simulink model "LTI_equivalente"  (R2023a)
settings: Solver=VariableStepAuto  StartTime=0.0  StopTime=1  RelTol=1e-3
undefined symbols (not defined in the file or in its folder): b_eq, Cts, J_eq, k_l, lambda, Lq, Pp, r, Rs_ref, Rts
libraries: SignalEditorBlockLib x3
settings Model: Creator=tobip  LastModifiedBy=tobip

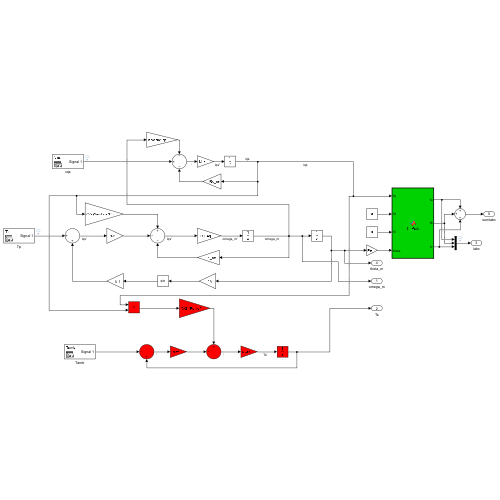
[thumbnail: Simulink's stored preview of the top-level diagram]
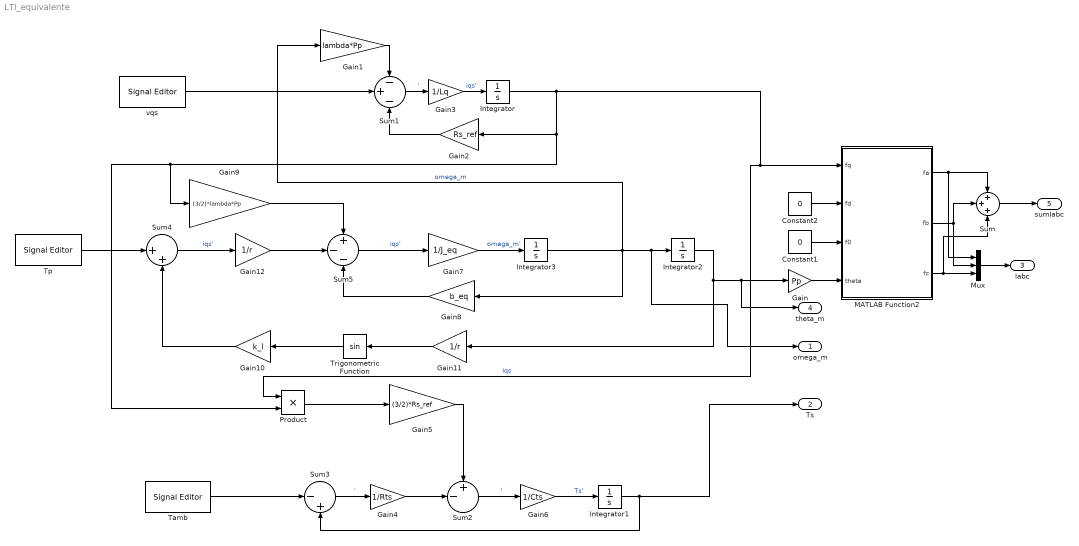
== system LTI_equivalente ==
  Constant1 : Constant  Value=0
  Constant2 : Constant  Value=0
  Gain : Gain  Gain=Pp
  Gain1 : Gain  Gain=lambda*Pp
  Gain10 : Gain  Gain=k_l
  Gain11 : Gain  Gain=1/r
  Gain12 : Gain  Gain=1/r
  Gain2 : Gain  Gain=Rs_ref
  Gain3 : Gain  Gain=1/Lq
  Gain4 : Gain  Gain=1/Rts
  Gain5 : Gain  Gain=(3/2)*Rs_ref
  Gain6 : Gain  Gain=1/Cts
  Gain7 : Gain  Gain=1/J_eq
  Gain8 : Gain  Gain=b_eq
  Gain9 : Gain  Gain=(3/2)*lambda*Pp
  Integrator{,1..3} (4 alike) : Integrator
  MATLAB Function2 : MATLAB Function  TreatAsAtomicUnit=on
  Mux : Mux  Inputs=3
  Product : Product
  Sum : Sum  Inputs=+++
  Sum1 : Sum  Inputs=-+-
  Sum2 : Sum  Inputs=+-|
  Sum3 : Sum  Inputs=|-+
  Sum4 : Sum  Inputs=|++
  Sum5 : Sum  Inputs=+--
  Tamb : SignalEditorBlockLib/Signal Editor  FileName=senal_Tamb.mat  ActiveScenario=Tamb  ActiveSignal=Constant  IsBus=off  OutputBusObjectStr=Bus: BusObject  SampleTime=0  Interpolate=off  ZeroCross=off  OutputAfterFinalValue=Setting to zero  Unit=inherit  PreserveSignalName=on  ApplySigPropsToAllScenarios=on
  Tp : SignalEditorBlockLib/Signal Editor  FileName=senal_Tp.mat  ActiveScenario=Tp  ActiveSignal=Pulse  IsBus=off  OutputBusObjectStr=Bus: BusObject  SampleTime=0  Interpolate=off  ZeroCross=off  OutputAfterFinalValue=Setting to zero  Unit=inherit  PreserveSignalName=on  ApplySigPropsToAllScenarios=on
  Trigonometric Function : Trigonometry
  vqs : SignalEditorBlockLib/Signal Editor  FileName=senal_vqs.mat  ActiveScenario=Vqs  ActiveSignal=Pulse  IsBus=off  OutputBusObjectStr=Bus: BusObject  SampleTime=0  Interpolate=off  ZeroCross=off  OutputAfterFinalValue=Setting to zero  Unit=inherit  PreserveSignalName=on  ApplySigPropsToAllScenarios=on
  omega_m : Outport
  Ts : Outport  Port=2
  Iabc : Outport  Port=3
  theta_m : Outport  Port=4
  sumIabc : Outport  Port=5
  wires:
  Integrator1/1 -> Ts/1, Sum3/2
  Integrator2/1 -> Gain/1, theta_m/1, Gain11/1
  Constant1/1 -> MATLAB Function2/3(f0)
  Gain/1 -> MATLAB Function2/4(theta)
  MATLAB Function2/1(fa) -> Sum/1, Mux/1
  MATLAB Function2/2(fb) -> Sum/2, Mux/2
  MATLAB Function2/3(fc) -> Mux/3, Sum/3
  Mux/1 -> Iabc/1
  Sum/1 -> sumIabc/1
  Constant2/1 -> MATLAB Function2/2(fd)
  Integrator/1 -> Gain2/1, Product/2, Gain9/1, Product/1, MATLAB Function2/1(fq)  "iqs"
  Gain1/1 -> Sum1/1
  vqs/1 -> Sum1/2
  Gain2/1 -> Sum1/3
  Sum1/1 -> Gain3/1  "'"
  Gain3/1 -> Integrator/1  "iqs'"
  Product/1 -> Gain5/1
  Tamb/1 -> Sum3/1
  Sum3/1 -> Gain4/1  "'"
  Sum2/1 -> Gain6/1  "'"
  Gain6/1 -> Integrator1/1  "Ts'"
  Gain4/1 -> Sum2/2
  Gain5/1 -> Sum2/1
  Gain11/1 -> Trigonometric Function/1
  Gain12/1 -> Sum5/2
  Gain10/1 -> Sum4/2
  Sum5/1 -> Gain7/1  "iqs'"
  Trigonometric Function/1 -> Gain10/1
  Sum4/1 -> Gain12/1  "iqs'"
  Tp/1 -> Sum4/1
  Gain7/1 -> Integrator3/1  "omega_m'"
  Integrator3/1 -> Gain1/1, Gain8/1, omega_m/1, Integrator2/1  "omega_m"
  Gain9/1 -> Sum5/1
  Gain8/1 -> Sum5/3

== matlab function LTI_equivalente/MATLAB Function2 ==
  data: fq input; fa output size=1; fd input; f0 input; theta input; fb output size=1; fc output size=1
function [fa,fb,fc] = TI_Park(fq,fd,f0,theta)

f = [     cos(theta)              sin(theta)         1;
       cos(theta - (2*pi)/3)   sin(theta - (2*pi)/3)   1;
       cos(theta + (2*pi)/3)   sin(theta + (2*pi)/3)   1];

resultados = f*[fq;fd;f0];
fa = resultados(1);
fb = resultados(2);
fc = resultados(3);
